simulink model "pd_control_test"  (R2016b)
settings: Solver=VariableStepAuto  StartTime=0.0  StopTime=100  RelTol=1e-3
libraries: dynamics_lib x1, environment_lib x1, pd_control_lib x1, RW_assembly_simple_lib x1
settings Model: Creator=taylorreynolds  LastModifiedBy=Taylor

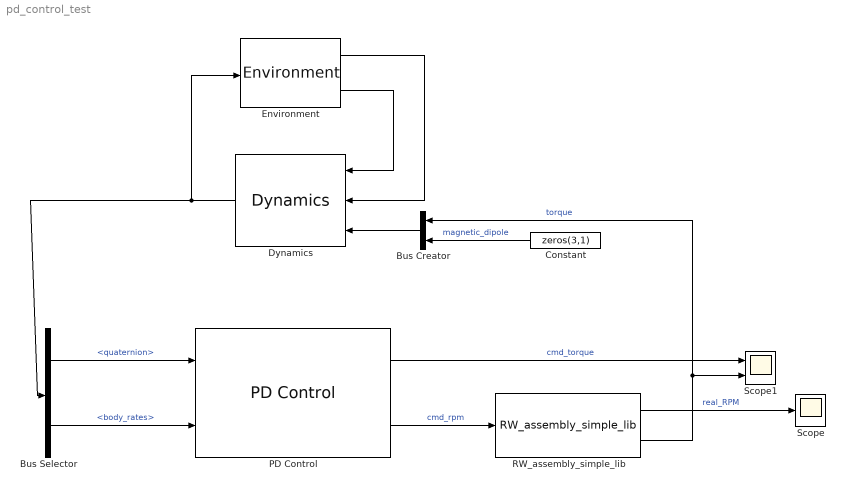
== system pd_control_test ==
  Bus Creator : BusCreator  Inputs=2
  Bus Selector : BusSelector  OutputSignals=quaternion,body_rates
  Constant : Constant  Value=zeros(3,1)
  Dynamics : dynamics_lib/Dynamics
  Environment : environment_lib/Environment
  PD Control : pd_control_lib/PD Control
  RW_assembly_simple_lib : RW_assembly_simple_lib/RW_assembly_simple_lib  natural_frequency=100  damping_ratio=1  max_rate=100
  Scope : Scope
  Scope1 : Scope  NumInputPorts=2
  wires:
  Environment/2 -> Dynamics/1
  Environment/1 -> Dynamics/2
  Dynamics/1 -> Environment/1, Bus Selector/1
  Bus Selector/2 -> PD Control/2  "<body_rates>"
  Bus Selector/1 -> PD Control/1  "<quaternion>"
  Bus Creator/1 -> Dynamics/3
  Constant/1 -> Bus Creator/2  "magnetic_dipole"
  PD Control/2 -> RW_assembly_simple_lib/1  "cmd_rpm"
  RW_assembly_simple_lib/2 -> Bus Creator/1, Scope1/2  "torque"
  PD Control/1 -> Scope1/1  "cmd_torque"
  RW_assembly_simple_lib/1 -> Scope/1  "real_RPM"
